simulink model "gate_V25_2016a"  (R2016a)
settings: Solver=FixedStepAuto  StartTime=0.0  StopTime=100  FixedStep=0.001  RelTol=1e-3
values from neighbouring files (symbols this model uses):
  CLOSE_CHAR = CHAR_STAR    (= 42)    [GateParameter.m]
  CLOSE_SIDE_VALUE = 2.95*oneSec    (= 2950)    [GateParameter.m]
  CLOSED = 12    [GateParameter.m]
  CLOSING = 13    [GateParameter.m]
  NO_PASS_ASSIG = 6    [GateParameter.m]
  OPEN = 14    [GateParameter.m]
  OPEN_CHAR = CHAR_HASH    (= 35)    [GateParameter.m]
  OPEN_SIDE_VALUE = 3*oneSec    (= 3000)    [GateParameter.m]
  OPEN_TIMEOUT = 60*oneSec    (= 60000)    [GateParameter.m]
  OPENING = 11    [GateParameter.m]
  OPENING_ACTIVE = 1    [GateParameter.m]
  PASS_ASSIGNED = 7    [GateParameter.m]
  PASS_INCOMPLETE = 8    [GateParameter.m]
  PASS_TIMEOUT = 10*oneSec    (= 10000)    [GateParameter.m]
  PASSWORD_VERIFIED = 5    [GateParameter.m]
  TIMEOUT = 9    [GateParameter.m]
  WRONG_PASSWORD = 2    [GateParameter.m]
undefined symbols (not defined in the file or in its folder): sigbuilder_block
libraries: simulink x9, arduinolib x4
(part 2 of 3)

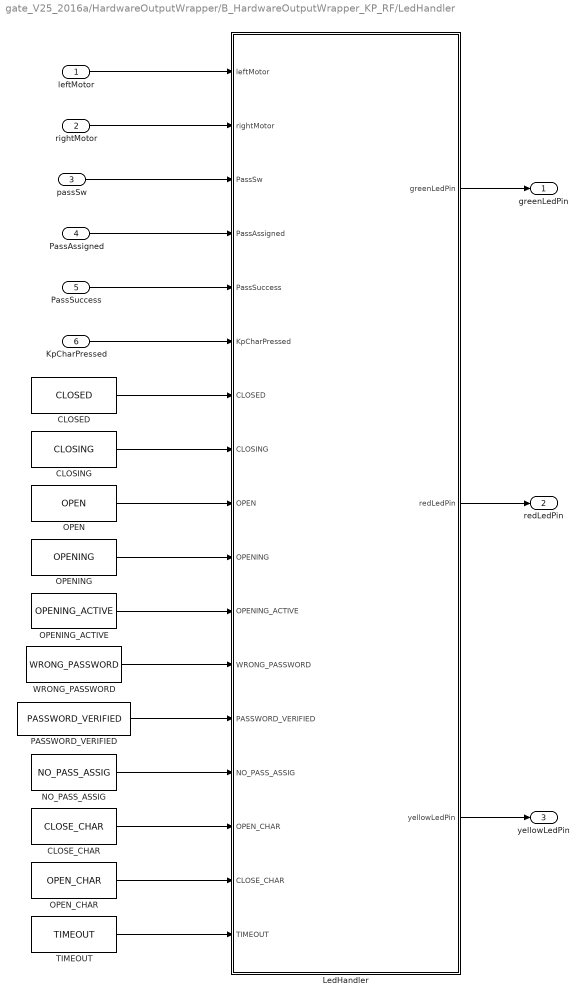
== system gate_V25_2016a/HardwareOutputWrapper/B_HardwareOutputWrapper_KP_RF/LedHandler ==
  leftMotor : Inport
  rightMotor : Inport  Port=2
  passSw : Inport  Port=3
  PassAssigned : Inport  Port=4
  PassSuccess : Inport  Port=5
  KpCharPressed : Inport  Port=6
  CLOSED : Constant  Value=CLOSED  SampleTime=-1
  CLOSE_CHAR : Constant  Value=CLOSE_CHAR  SampleTime=-1
  CLOSING : Constant  Value=CLOSING  SampleTime=-1
  LedHandler : Stateflow chart  TreatAsAtomicUnit=on
      settings: PermitHierarchicalResolution=ParametersOnly
  NO_PASS_ASSIG : Constant  Value=NO_PASS_ASSIG  SampleTime=-1
  OPEN : Constant  Value=OPEN  SampleTime=-1
  OPENING : Constant  Value=OPENING  SampleTime=-1
  OPENING_ACTIVE : Constant  Value=OPENING_ACTIVE  SampleTime=-1
  OPEN_CHAR : Constant  Value=OPEN_CHAR  SampleTime=-1
  PASSWORD_VERIFIED : Constant  Value=PASSWORD_VERIFIED  SampleTime=-1
  TIMEOUT : Constant  Value=TIMEOUT  SampleTime=-1
  WRONG_PASSWORD : Constant  Value=WRONG_PASSWORD  SampleTime=-1
  greenLedPin : Outport
  redLedPin : Outport  Port=2
  yellowLedPin : Outport  Port=3
  wires:
  TIMEOUT/1 -> LedHandler/17(TIMEOUT)
  OPEN_CHAR/1 -> LedHandler/16(CLOSE_CHAR)
  CLOSE_CHAR/1 -> LedHandler/15(OPEN_CHAR)
  KpCharPressed/1 -> LedHandler/6(KpCharPressed)
  NO_PASS_ASSIG/1 -> LedHandler/14(NO_PASS_ASSIG)
  PASSWORD_VERIFIED/1 -> LedHandler/13(PASSWORD_VERIFIED)
  WRONG_PASSWORD/1 -> LedHandler/12(WRONG_PASSWORD)
  OPENING_ACTIVE/1 -> LedHandler/11(OPENING_ACTIVE)
  CLOSED/1 -> LedHandler/7(CLOSED)
  CLOSING/1 -> LedHandler/8(CLOSING)
  OPEN/1 -> LedHandler/9(OPEN)
  OPENING/1 -> LedHandler/10(OPENING)
  PassSuccess/1 -> LedHandler/5(PassSuccess)
  PassAssigned/1 -> LedHandler/4(PassAssigned)
  passSw/1 -> LedHandler/3(PassSw)
  LedHandler/3(yellowLedPin) -> yellowLedPin/1
  LedHandler/2(redLedPin) -> redLedPin/1
  LedHandler/1(greenLedPin) -> greenLedPin/1
  rightMotor/1 -> LedHandler/2(rightMotor)
  leftMotor/1 -> LedHandler/1(leftMotor)

== system gate_V25_2016a/HardwareOutputWrapper/B_HardwareOutputWrapper_KP_RF/MotorHandler ==
  leftMotor : Inport
  rightMotor : Inport  Port=2
  CLOSED : Constant  Value=CLOSED  SampleTime=-1
  CLOSING : Constant  Value=CLOSING  SampleTime=-1
  MotorsHandler : Stateflow chart  TreatAsAtomicUnit=on
      settings: PermitHierarchicalResolution=ParametersOnly
  OPEN : Constant  Value=OPEN  SampleTime=-1
  OPENING : Constant  Value=OPENING  SampleTime=-1
  Unit Delay : UnitDelay  SampleTime=-1
  Unit Delay1 : UnitDelay  SampleTime=-1
  LeftPin : Outport
  ComPin : Outport  Port=2
  RightPin : Outport  Port=3
  wires:
  MotorsHandler/3(RightPin) -> RightPin/1
  MotorsHandler/2(ComPin) -> ComPin/1
  MotorsHandler/1(LeftPin) -> LeftPin/1
  OPENING/1 -> MotorsHandler/8(OPENING)
  OPEN/1 -> MotorsHandler/7(OPEN)
  CLOSING/1 -> MotorsHandler/6(CLOSING)
  CLOSED/1 -> MotorsHandler/5(CLOSED)
  Unit Delay1/1 -> MotorsHandler/4(oldRight)
  rightMotor/1 -> MotorsHandler/3(rightMotor), Unit Delay1/1
  Unit Delay/1 -> MotorsHandler/2(oldLeft)
  leftMotor/1 -> MotorsHandler/1(leftMotor), Unit Delay/1

== system gate_V25_2016a/HardwareOutputWrapper/C_HardwareOutputWrapper_RF/BulbHandler ==
  bulb : Inport
  bulbPin : Outport
  wires:
  bulb/1 -> bulbPin/1

== system gate_V25_2016a/HardwareOutputWrapper/C_HardwareOutputWrapper_RF/MotorHandler ==
  leftMotor : Inport
  rightMotor : Inport  Port=2
  CLOSED : Constant  Value=CLOSED  SampleTime=-1
  CLOSING : Constant  Value=CLOSING  SampleTime=-1
  MotorsHandler : Stateflow chart  TreatAsAtomicUnit=on
      settings: PermitHierarchicalResolution=ParametersOnly
  OPEN : Constant  Value=OPEN  SampleTime=-1
  OPENING : Constant  Value=OPENING  SampleTime=-1
  Unit Delay : UnitDelay  SampleTime=-1
  Unit Delay1 : UnitDelay  SampleTime=-1
  LeftPin : Outport
  ComPin : Outport  Port=2
  RightPin : Outport  Port=3
  wires:
  leftMotor/1 -> Unit Delay/1, MotorsHandler/1(leftMotor)
  Unit Delay/1 -> MotorsHandler/2(oldLeft)
  rightMotor/1 -> Unit Delay1/1, MotorsHandler/3(rightMotor)
  Unit Delay1/1 -> MotorsHandler/4(oldRight)
  CLOSED/1 -> MotorsHandler/5(CLOSED)
  CLOSING/1 -> MotorsHandler/6(CLOSING)
  OPEN/1 -> MotorsHandler/7(OPEN)
  OPENING/1 -> MotorsHandler/8(OPENING)
  MotorsHandler/1(LeftPin) -> LeftPin/1
  MotorsHandler/2(ComPin) -> ComPin/1
  MotorsHandler/3(RightPin) -> RightPin/1

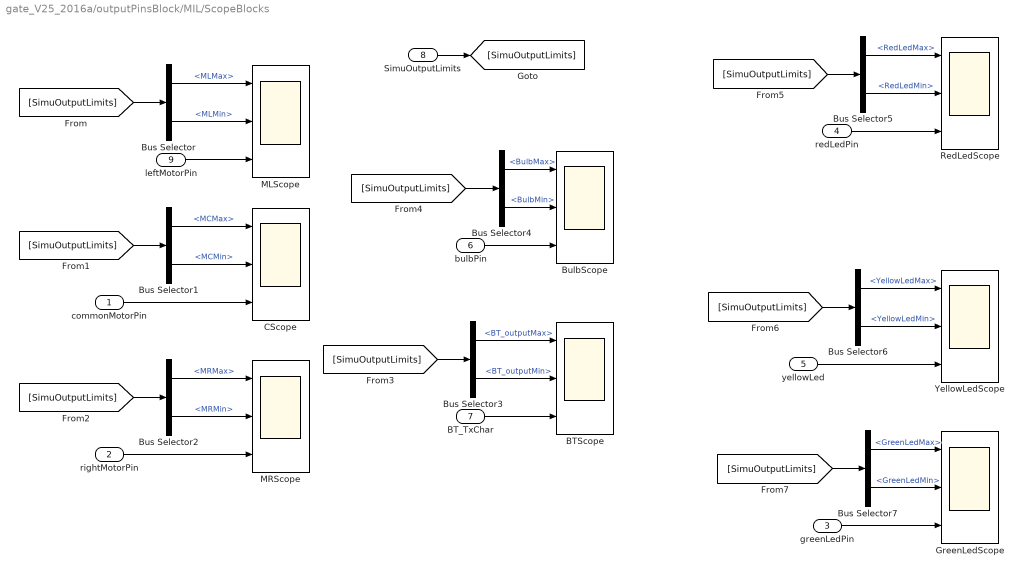
== system gate_V25_2016a/outputPinsBlock/MIL/ScopeBlocks ==
  commonMotorPin : Inport
  rightMotorPin : Inport  Port=2
  greenLedPin : Inport  Port=3
  redLedPin : Inport  Port=4
  yellowLed : Inport  Port=5
  bulbPin : Inport  Port=6
  BT_TxChar : Inport  Port=7
  SimuOutputLimits : Inport  Port=8
  leftMotorPin : Inport  Port=9
  BTScope : Scope  NumInputPorts=3
  BulbScope : Scope  NumInputPorts=3
  Bus Selector : BusSelector  OutputSignals=MLMax,MLMin
  Bus Selector1 : BusSelector  OutputSignals=MCMax,MCMin
  Bus Selector2 : BusSelector  OutputSignals=MRMax,MRMin
  Bus Selector3 : BusSelector  OutputSignals=BT_outputMax,BT_outputMin
  Bus Selector4 : BusSelector  OutputSignals=BulbMax,BulbMin
  Bus Selector5 : BusSelector  OutputSignals=RedLedMax,RedLedMin
  Bus Selector6 : BusSelector  OutputSignals=YellowLedMax,YellowLedMin
  Bus Selector7 : BusSelector  OutputSignals=GreenLedMax,GreenLedMin
  CScope : Scope  NumInputPorts=3
  GreenLedScope : Scope  NumInputPorts=3
  MLScope : Scope  NumInputPorts=3
  MRScope : Scope  NumInputPorts=3
  RedLedScope : Scope  NumInputPorts=3
  YellowLedScope : Scope  NumInputPorts=3
  wires:
  rightMotorPin/1 -> MRScope/3
  commonMotorPin/1 -> CScope/3
  bulbPin/1 -> BulbScope/3
  greenLedPin/1 -> GreenLedScope/3
  yellowLed/1 -> YellowLedScope/3
  redLedPin/1 -> RedLedScope/3
  BT_TxChar/1 -> BTScope/3
  SimuOutputLimits/1 -> [SimuOutputLimits]
  [SimuOutputLimits] -> Bus Selector/1
  leftMotorPin/1 -> MLScope/3
  Bus Selector/1 -> MLScope/1  "<MLMax>"
  Bus Selector/2 -> MLScope/2  "<MLMin>"
  [SimuOutputLimits] -> Bus Selector1/1
  Bus Selector1/1 -> CScope/1  "<MCMax>"
  Bus Selector1/2 -> CScope/2  "<MCMin>"
  [SimuOutputLimits] -> Bus Selector2/1
  Bus Selector2/1 -> MRScope/1  "<MRMax>"
  Bus Selector2/2 -> MRScope/2  "<MRMin>"
  [SimuOutputLimits] -> Bus Selector3/1
  Bus Selector3/1 -> BTScope/1  "<BT_outputMax>"
  Bus Selector3/2 -> BTScope/2  "<BT_outputMin>"
  [SimuOutputLimits] -> Bus Selector4/1
  Bus Selector4/1 -> BulbScope/1  "<BulbMax>"
  Bus Selector4/2 -> BulbScope/2  "<BulbMin>"
  [SimuOutputLimits] -> Bus Selector5/1
  Bus Selector5/1 -> RedLedScope/1  "<RedLedMax>"
  Bus Selector5/2 -> RedLedScope/2  "<RedLedMin>"
  [SimuOutputLimits] -> Bus Selector6/1
  Bus Selector6/1 -> YellowLedScope/1  "<YellowLedMax>"
  Bus Selector6/2 -> YellowLedScope/2  "<YellowLedMin>"
  [SimuOutputLimits] -> Bus Selector7/1
  Bus Selector7/1 -> GreenLedScope/1  "<GreenLedMax>"
  Bus Selector7/2 -> GreenLedScope/2  "<GreenLedMin>"

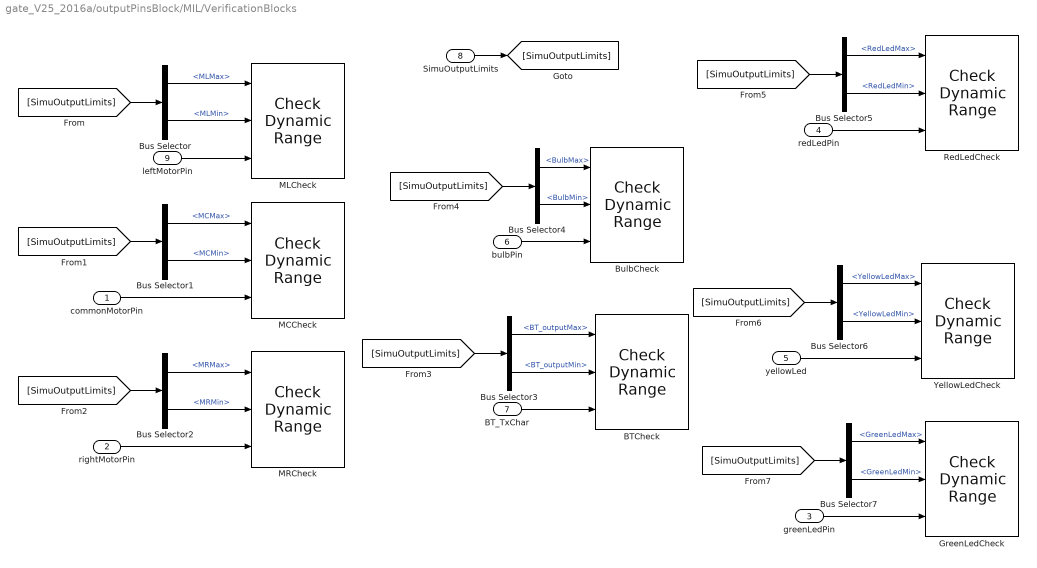
== system gate_V25_2016a/outputPinsBlock/MIL/VerificationBlocks  ==
  commonMotorPin : Inport
  rightMotorPin : Inport  Port=2
  greenLedPin : Inport  Port=3
  redLedPin : Inport  Port=4
  yellowLed : Inport  Port=5
  bulbPin : Inport  Port=6
  BT_TxChar : Inport  Port=7
  SimuOutputLimits : Inport  Port=8
  leftMotorPin : Inport  Port=9
  BTCheck : simulink/Model Verification/Check  Dynamic Range  Description=min < sig < max  enabled=on  stopWhenAssertionFail=on  export=off  icon=graphic
  BulbCheck : simulink/Model Verification/Check  Dynamic Range  Description=min < sig < max  enabled=on  stopWhenAssertionFail=on  export=off  icon=graphic
  Bus Selector : BusSelector  OutputSignals=MLMax,MLMin
  Bus Selector1 : BusSelector  OutputSignals=MCMax,MCMin
  Bus Selector2 : BusSelector  OutputSignals=MRMax,MRMin
  Bus Selector3 : BusSelector  OutputSignals=BT_outputMax,BT_outputMin
  Bus Selector4 : BusSelector  OutputSignals=BulbMax,BulbMin
  Bus Selector5 : BusSelector  OutputSignals=RedLedMax,RedLedMin
  Bus Selector6 : BusSelector  OutputSignals=YellowLedMax,YellowLedMin
  Bus Selector7 : BusSelector  OutputSignals=GreenLedMax,GreenLedMin
  GreenLedCheck : simulink/Model Verification/Check  Dynamic Range  Description=min < sig < max  enabled=on  stopWhenAssertionFail=on  export=off  icon=graphic
  MCCheck : simulink/Model Verification/Check  Dynamic Range  Description=min < sig < max  enabled=on  stopWhenAssertionFail=on  export=off  icon=graphic
  MLCheck : simulink/Model Verification/Check  Dynamic Range  Description=min < sig < max  enabled=on  stopWhenAssertionFail=on  export=off  icon=graphic
  MRCheck : simulink/Model Verification/Check  Dynamic Range  Description=min < sig < max  enabled=on  stopWhenAssertionFail=on  export=off  icon=graphic
  RedLedCheck : simulink/Model Verification/Check  Dynamic Range  Description=min < sig < max  enabled=on  stopWhenAssertionFail=on  export=off  icon=graphic
  YellowLedCheck : simulink/Model Verification/Check  Dynamic Range  Description=min < sig < max  enabled=on  stopWhenAssertionFail=on  export=off  icon=graphic
  wires:
  rightMotorPin/1 -> MRCheck/3
  commonMotorPin/1 -> MCCheck/3
  bulbPin/1 -> BulbCheck/3
  greenLedPin/1 -> GreenLedCheck/3
  yellowLed/1 -> YellowLedCheck/3
  redLedPin/1 -> RedLedCheck/3
  BT_TxChar/1 -> BTCheck/3
  SimuOutputLimits/1 -> [SimuOutputLimits]
  [SimuOutputLimits] -> Bus Selector/1
  leftMotorPin/1 -> MLCheck/3
  Bus Selector/1 -> MLCheck/1  "<MLMax>"
  Bus Selector/2 -> MLCheck/2  "<MLMin>"
  [SimuOutputLimits] -> Bus Selector1/1
  Bus Selector1/1 -> MCCheck/1  "<MCMax>"
  Bus Selector1/2 -> MCCheck/2  "<MCMin>"
  [SimuOutputLimits] -> Bus Selector2/1
  Bus Selector2/1 -> MRCheck/1  "<MRMax>"
  Bus Selector2/2 -> MRCheck/2  "<MRMin>"
  [SimuOutputLimits] -> Bus Selector3/1
  Bus Selector3/1 -> BTCheck/1  "<BT_outputMax>"
  Bus Selector3/2 -> BTCheck/2  "<BT_outputMin>"
  [SimuOutputLimits] -> Bus Selector4/1
  Bus Selector4/1 -> BulbCheck/1  "<BulbMax>"
  Bus Selector4/2 -> BulbCheck/2  "<BulbMin>"
  [SimuOutputLimits] -> Bus Selector5/1
  Bus Selector5/1 -> RedLedCheck/1  "<RedLedMax>"
  Bus Selector5/2 -> RedLedCheck/2  "<RedLedMin>"
  [SimuOutputLimits] -> Bus Selector6/1
  Bus Selector6/1 -> YellowLedCheck/1  "<YellowLedMax>"
  Bus Selector6/2 -> YellowLedCheck/2  "<YellowLedMin>"
  [SimuOutputLimits] -> Bus Selector7/1
  Bus Selector7/1 -> GreenLedCheck/1  "<GreenLedMax>"
  Bus Selector7/2 -> GreenLedCheck/2  "<GreenLedMin>"

== stateflow chart gate_V25_2016a/GateLogic/A_Variant_BT_KP_RF/GateLogicStatemachine ==
  state opening
    entry:
    bulb = true;
    state openLeftSide
      entry:
      leftMotor = OPENING;
      openSideDelay = 0;
      during:
      openSideDelay++;
    state openRightSide
      entry:
      rightMotor = OPENING;
    (default) -> openLeftSide
    openLeftSide -> openRightSide : [openSideDelay == OPEN_SIDE_VALUE]
  state init
    entry:
    passSuccess = NO_PASS_ASSIG;
    gotoReady = false;
    bulb = 0;
    leftMotor = CLOSED;
    rightMotor = CLOSED;
    state AssignPass
      entry:
      counter = 0;
      state addToPass
        entry:
        password[counter] = KpCharPressed;
      state MonitoringNumber
      state PassAssigned
        entry:
        gotoReady = true;
      (junction 259) -> addToPass : [KpCharPressed != 0]
      MonitoringNumber -> (junction 259) [order 1] : [hasChanged(KpCharPressed)]
      (default) -> MonitoringNumber
      addToPass -> MonitoringNumber [order 1] : [counter < 5]/counter++;
      MonitoringNumber -> PassAssigned [order 2] : [RfOpen == true]
      addToPass -> PassAssigned [order 2] : [counter == 5]
          | / passAssigned = true;...
          | passSuccess = PASS_ASSIGNED;
    state idle
      entry:
      passAssigned = false;
    state PassAssignedPreviously
      entry:
      password[0] = passwordIn[0];
      password[1] = passwordIn[1];
      password[2] = passwordIn[2];
      password[3] = passwordIn[3];
      password[4] = passwordIn[4];
      password[5] = passwordIn[5];
      passAssigned = passAssignedIn;
      gotoReady = true;
    (default) -> idle
    idle -> AssignPass [order 1] : [passSwitch==true]
    idle -> PassAssignedPreviously [order 2] : [passAssignedIn]
    AssignPass -> idle : [passSwitch==false]
  state ready
    entry:
    bulb = false;
    leftMotor = CLOSED;
    rightMotor = CLOSED;
    openingActive = 0;
    state BTPassHandler
      state monitorBtnPressed
      state btnPressed
        entry:
        trialPass[counter] = BtCharReceived;
      state initTrailPass
        entry:
        initCounter = 1;
        state initiatePass
          entry:
          trialPass[initCounter] = 0;
        (junction 295) -> ready.BTPassHandler.initTrailPass.initiatePass
        (default) -> (junction 295)
        ready.BTPassHandler.initTrailPass.initiatePass -> (junction 295) : [initCounter < 5]...
            | /initCounter++;
      state verifyPass
        (default) -> (junction 301)
        (junction 301) -> (junction 302) [order 1] : [trialPass[0] != password[0]]
        (junction 301) -> (junction 303) [order 2]
        (junction 302) -> (junction 319) : {passSuccess = WRONG_PASSWORD;}
        (junction 303) -> (junction 304) [order 1] : [trialPass[1] != password[1]]
        (junction 303) -> (junction 305) [order 2]
        (junction 304) -> (junction 318) : {passSuccess = WRONG_PASSWORD;}
        (junction 305) -> (junction 306) [order 1] : [trialPass[2] != password[2]]
        (junction 305) -> (junction 307) [order 2]
        (junction 306) -> (junction 317) : {passSuccess = WRONG_PASSWORD;}
        (junction 307) -> (junction 308) [order 1] : [trialPass[3] != password[3]]
        (junction 307) -> (junction 309) [order 2]
        (junction 308) -> (junction 316) : {passSuccess = WRONG_PASSWORD;}
        (junction 309) -> (junction 310) [order 1] : [trialPass[4] != password[4]]
        (junction 309) -> (junction 311) [order 2]
        (junction 310) -> (junction 315) : {passSuccess = WRONG_PASSWORD;}
        (junction 311) -> (junction 312) [order 1] : [trialPass[5] != password[5]]
        (junction 311) -> (junction 313) [order 2] : {passSuccess = PASSWORD_VERIFIED;}
        (junction 312) -> (junction 314) : {passSuccess = WRONG_PASSWORD;}
        (junction 314) -> (junction 313)
        (junction 315) -> (junction 314)
        (junction 316) -> (junction 315)
        (junction 317) -> (junction 316)
        (junction 318) -> (junction 317)
        (junction 319) -> (junction 318)
        (junction 313) -> (junction 320)
      (default) -> ready.BTPassHandler.initTrailPass
      ready.BTPassHandler.monitorBtnPressed -> (junction 277) : [hasChanged...
          | (BtCharReceived)]
      (junction 277) -> ready.BTPassHandler.btnPressed : [BtCharReceived != 0]/{counter++;}
      ready.BTPassHandler.initTrailPass -> ready.BTPassHandler.monitorBtnPressed : [initCounter == 5]...
          | /{counter = 0;}
      ready.BTPassHandler.btnPressed -> ready.BTPassHandler.monitorBtnPressed [order 1] : [counter < 5]
      (junction 279) -> ready.BTPassHandler.initTrailPass
      ready.BTPassHandler.btnPressed -> ready.BTPassHandler.verifyPass [order 2] : [counter >= 5]
      ready.BTPassHandler.verifyPass -> (junction 279) : [(passSuccess == PASSWORD_VERIFIED)]
          | / {openingActive = OPENING_ACTIVE;}
    state openingGate
    state MonitorInput
      entry:
      passTimer = 0;
    state KpPassHandler
      du:
      passTimer++;
      state monitorBtnPressed
      state btnPressed
        entry:
        trialPass[counter] = KpCharPressed;
      state initTrailPass
        entry:
        initCounter = 1;
        state initiatePass
          entry:
          trialPass[initCounter] = 0;
        (junction 269) -> ready.KpPassHandler.initTrailPass.initiatePass
        (default) -> (junction 269)
        ready.KpPassHandler.initTrailPass.initiatePass -> (junction 269) : [initCounter < 5]...
            | /initCounter++;
      state verifyPass
        (default) -> (junction 115)
        (junction 115) -> (junction 116) [order 1] : [trialPass[0] != password[0]]
        (junction 115) -> (junction 119) [order 2]
        (junction 116) -> (junction 118) : {passSuccess = WRONG_PASSWORD;}
        (junction 119) -> (junction 122) [order 1] : [trialPass[1] != password[1]]
        (junction 119) -> (junction 120) [order 2]
        (junction 122) -> (junction 121) : {passSuccess = WRONG_PASSWORD;}
        (junction 120) -> (junction 144) [order 1] : [trialPass[2] != password[2]]
        (junction 120) -> (junction 143) [order 2]
        (junction 144) -> (junction 168) : {passSuccess = WRONG_PASSWORD;}
        (junction 143) -> (junction 149) [order 1] : [trialPass[3] != password[3]]
        (junction 143) -> (junction 153) [order 2]
        (junction 149) -> (junction 169) : {passSuccess = WRONG_PASSWORD;}
        (junction 153) -> (junction 156) [order 1] : [trialPass[4] != password[4]]
        (junction 153) -> (junction 157) [order 2]
        (junction 156) -> (junction 170) : {passSuccess = WRONG_PASSWORD;}
        (junction 157) -> (junction 158) [order 1] : [trialPass[5] != password[5]]
        (junction 157) -> (junction 164) [order 2] : {passSuccess = PASSWORD_VERIFIED;}
        (junction 158) -> (junction 171) : {passSuccess = WRONG_PASSWORD;}
        (junction 171) -> (junction 164)
        (junction 170) -> (junction 171)
        (junction 169) -> (junction 170)
        (junction 168) -> (junction 169)
        (junction 121) -> (junction 168)
        (junction 118) -> (junction 121)
        (junction 164) -> (junction 165)
      (default) -> ready.KpPassHandler.initTrailPass
      ready.KpPassHandler.monitorBtnPressed -> (junction 263) : [hasChanged...
          | (KpCharPressed)]
      (junction 263) -> ready.KpPassHandler.btnPressed : [KpCharPressed != 0]/{counter++;}
      ready.KpPassHandler.initTrailPass -> ready.KpPassHandler.monitorBtnPressed : [initCounter == 5]...
          | /{counter = 0;}
      ready.KpPassHandler.btnPressed -> ready.KpPassHandler.monitorBtnPressed [order 1] : [counter < 5]
      (junction 262) -> ready.KpPassHandler.initTrailPass : [(KpCharPressed == OPEN_CHAR)...
          |  && (KpCharPressed != 0)]...
          |  / {openingActive = OPENING_ACTIVE;}
      ready.KpPassHandler.btnPressed -> ready.KpPassHandler.verifyPass [order 2] : [counter >= 5]
      ready.KpPassHandler.verifyPass -> (junction 262) : [hasChanged(KpCharPressed) && (passSuccess == PASSWORD_VERIFIED)]
    (junction 350) -> BTPassHandler : [(BtCharReceived != 0) ...
        | && passAssigned]
        | /passSuccess = PASS_INCOMPLETE;...
        | trialPass[0] = BtCharReceived;
    MonitorInput -> (junction 350) [order 3] : [hasChanged...
        | (BtCharReceived)]
    BTPassHandler -> openingGate [order 2] : [openingActive == OPENING_ACTIVE]
    BTPassHandler -> MonitorInput [order 1] : [passSuccess == WRONG_PASSWORD]
    MonitorInput -> openingGate [order 1] : [RfOpen]/{openingActive = OPENING_ACTIVE;}
    (default) -> MonitorInput
    KpPassHandler -> MonitorInput [order 3] : [(passTimer == PASS_TIMEOUT)]
        | /passSuccess = TIMEOUT;
    KpPassHandler -> openingGate [order 1] : [openingActive == OPENING_ACTIVE]
    MonitorInput -> (junction 260) [order 2] : [hasChanged...
        | (KpCharPressed)]
    KpPassHandler -> MonitorInput [order 2] : [(passSuccess == WRONG_PASSWORD)]
    (junction 260) -> KpPassHandler : [(KpCharPressed != 0) ...
        | &&(KpCharPressed != OPEN_CHAR)...
        | &&(KpCharPressed != CLOSE_CHAR)...
        | && passAssigned]
        | /passSuccess = PASS_INCOMPLETE;...
        | trialPass[0] = KpCharPressed;
  state closing
    state closingRightSide
      entry:
      rightMotor = CLOSING;
      closeSideDelay = 0;
      during:
      closeSideDelay++;
    state closingLeftSide
      entry:
      leftMotor = CLOSING;
    (default) -> closingRightSide
    closingRightSide -> closingLeftSide : [closeSideDelay == CLOSE_SIDE_VALUE]
  state open
    state gateOpen
      entry:
      closing_active = false;
      leftMotor = OPEN;
      rightMotor = OPEN;
      openTimer = 0;
      du:
      openTimer++;
    state closing
      entry:
      closing_active = true;
    (default) -> gateOpen
    gateOpen -> (junction 264) [order 1] : [hasChanged(KpCharPressed)]
    (junction 264) -> open.closing : [(KpCharPressed == CLOSE_CHAR)]
    gateOpen -> (junction 355) [order 3] : [hasChanged(BtCharReceived)]
    (junction 355) -> open.closing : [BtCharReceived == CLOSE_CHAR]
    gateOpen -> open.closing [order 2] : [RfClose]
    gateOpen -> open.closing [order 4] : [openTimer == OPEN_TIMEOUT]
  ready -> (junction 258) [order 1] : [hasChanged(passSwitch)]
  (junction 258) -> init : [passSwitch]
  (default) -> init
  init -> ready [order 1] : [gotoReady == true]
  ready -> opening [order 2] : [openingActive == OPENING_ACTIVE]
  init -> ready [order 2] : [RfOpen == true]
  closing -> ready : [(current_sensor == 0)...
      | &&(leftMotor == CLOSING)...
      | &&(rightMotor == CLOSING)]
  opening -> open : [(current_sensor == 0)...
      | && (leftMotor == OPENING)...
      | && (rightMotor == OPENING)]
  open -> closing : [closing_active == true]
  data: KpCharPressed input; RfOpen input; openingActive local uint8; passSwitch input; counter local uint8; closing_active local uint8; current_sensor input; initCounter local uint8; openSideDelay local uint16; leftMotor output uint8 =0; rightMotor output uint8 =0; bulb output boolean; RfClose input; closeSideDelay local uint16; BtCharReceived input; OPENING_ACTIVE input =2; WRONG_PASSWORD input =1; OPEN_SIDE_VALUE input =20; CLOSE_SIDE_VALUE input =20; OPEN_TIMEOUT input =999999; PASSWORD_VERIFIED input =3; CLOSE_CHAR input =12; OPEN_CHAR input; OPENING input =2; CLOSED input =1; CLOSING input =4; OPEN input =3; passAssigned output boolean; gotoReady local boolean; passSuccess output uint8 =0; NO_PASS_ASSIG input; PASS_ASSIGNED input; PASS_INCOMPLETE input; PASS_TIMEOUT input; passTimer local uint16; TIMEOUT input; openTimer local uint16; password output uint8 size=6; passwordIn input size=6; passAssignedIn input; trialPass output uint8 size=6

== stateflow chart gate_V25_2016a/HardwareOutputWrapper/A_HardwareOutputWrapper_BT_KP_RF/BT_TxHandler/BT_TxHandler ==
  state Idle
    entry:
    BT_TxChar = 0;
  state WrongPass
    entry:
    BT_TxChar = 119;
    counter = 0;
    du:
    counter++;
  state BtInput
  state sendClose
    entry:
    BT_TxChar = 99;
  state sendOpen
    entry:
    BT_TxChar = 98;
  state sendOpening
    entry:
    BT_TxChar = 97;
  (default) -> Idle
  Idle -> (junction 8) : [hasChanged(BTCharReceived)]
  (junction 8) -> BtInput : [BTCharReceived != 0]
  sendClose -> Idle : [leftMotor == CLOSED]
  WrongPass -> Idle : [counter >= 10]
  BtInput -> WrongPass [order 2] : [PassSuccess == WRONG_PASSWORD]
  BtInput -> sendOpening [order 1] : [leftMotor == OPENING]
  sendOpen -> sendClose : [rightMotor == CLOSING]
  sendOpening -> sendOpen : [rightMotor == OPEN]
  data: BTCharReceived input; leftMotor input; rightMotor input; BT_TxChar output uint8; PassSuccess input; CLOSED input; CLOSING input; OPEN input; OPENING input; WRONG_PASSWORD input; counter local uint8

== stateflow chart gate_V25_2016a/HardwareOutputWrapper/A_HardwareOutputWrapper_BT_KP_RF/LedHandler/LedHandler ==
  state AssigningPass
    en:
    counter = 0;
    state Start
      en:
      yellowLedPin = true;
      greenLedPin = false;
      redLedPin = false;
    state correctPassAssigned
      du:
      counter++;
    state incorrectPassAssigned
      du:
      counter++;
    (default) -> AssigningPass.Start
    AssigningPass.Start -> correctPassAssigned [order 1] : [PassAssigned == true]/greenLedPin = true;
    AssigningPass.Start -> incorrectPassAssigned [order 2] : [(PassSw == false) && (PassAssigned == false)]
        | /redLedPin = true;...
        | yellowLedPin = false;
    correctPassAssigned -> correctPassAssigned : [(hasChanged(PassSw)) ...
        | && (PassSw == false)]
        | /yellowLedPin = false;
  state EnteringPass
    en:
    counter = 0;
    state correctPass
      en:
      yellowLedPin = false;
      greenLedPin = true;
      redLedPin = false;
      du:
      counter++;
    state Start
    state IncorrectPass
      en:
      yellowLedPin = false;
      greenLedPin = false;
      redLedPin = true;
      du:
      counter++;
    EnteringPass.Start -> correctPass [order 1] : [PassSuccess == PASSWORD_VERIFIED]
    (default) -> EnteringPass.Start
    EnteringPass.Start -> IncorrectPass [order 2] : [(PassSuccess == TIMEOUT)...
        |  || (PassSuccess == WRONG_PASSWORD)]
  state Idle
    en:
    yellowLedPin = false;
    greenLedPin = false;
    redLedPin = false;
  state GateOn
    en:
    yellowLedPin = false;
    greenLedPin = true;
    redLedPin = false;
  (default) -> Idle
  EnteringPass -> Idle [order 2] : [PassSuccess == NO_PASS_ASSIG]
  Idle -> AssigningPass [order 1] : [PassSw == true]
  correctPass -> Idle : [counter >= 4800]
  AssigningPass -> Idle [order 1] : [(counter >= 4900)]
  Idle -> EnteringPass [order 2] : [(hasChanged(KpCharPressed)) ...
      | && (KpCharPressed != 0)...
      | && (KpCharPressed != OPEN_CHAR)...
      | && (KpCharPressed != CLOSE_CHAR)...
      | && (PassAssigned == true)]
      | /yellowLedPin = true;
  IncorrectPass -> Idle : [counter >= 4800]
  Idle -> GateOn [order 3] : [(leftMotor == OPENING)...
      |  || (leftMotor == OPEN)...
      |  || (leftMotor == CLOSING)]
  GateOn -> Idle : [leftMotor == CLOSED]
  EnteringPass -> GateOn [order 1] : [(leftMotor == OPENING)...
      | || (leftMotor == OPEN)...
      | || (leftMotor == CLOSING)]
  AssigningPass -> GateOn [order 2] : [(leftMotor == OPENING)...
      |  || (leftMotor == OPEN)...
      |  || (leftMotor == CLOSING)]
  data: leftMotor input; rightMotor input; greenLedPin output boolean =false; redLedPin output boolean =false; yellowLedPin output boolean =false; PassSw input; counter local uint16; PassAssigned input; PassSuccess input; KpCharPressed input; CLOSED input; CLOSING input; OPEN input; OPENING input; OPENING_ACTIVE input; WRONG_PASSWORD input; PASSWORD_VERIFIED input; NO_PASS_ASSIG input; OPEN_CHAR input; CLOSE_CHAR input; TIMEOUT input

== stateflow chart gate_V25_2016a/GateLogic/B_Variant_KP_RF/GateLogicStatemachine ==
  state opening
    entry:
    bulb = true;
    state openLeftSide
      entry:
      leftMotor = OPENING;
      openSideDelay = 0;
      during:
      openSideDelay++;
    state openRightSide
      entry:
      rightMotor = OPENING;
    (default) -> openLeftSide
    openLeftSide -> openRightSide : [openSideDelay == OPEN_SIDE_VALUE]
  state init
    entry:
    passSuccess = NO_PASS_ASSIG;
    gotoReady = false;
    bulb = 0;
    leftMotor = CLOSED;
    rightMotor = CLOSED;
    state AssignPass
      entry:
      counter = 0;
      password[0] = 0;
      password[1] = 0;
      password[2] = 0;
      password[3] = 0;
      password[4] = 0;
      password[5] = 0;
      state addToPass
        entry:
        password[counter] = KpCharPressed;
      state MonitoringNumber
      state PassAssigned
        entry:
        gotoReady = true;
      MonitoringNumber -> (junction 259) [order 1] : [hasChanged(KpCharPressed)]
      (junction 259) -> addToPass : [KpCharPressed != 0]
      (default) -> MonitoringNumber
      addToPass -> MonitoringNumber [order 1] : [counter < 5]/counter++;
      addToPass -> PassAssigned [order 2] : [counter == 5]
          | / passAssigned = true;...
          | passSuccess = PASS_ASSIGNED;
      MonitoringNumber -> PassAssigned [order 2] : [RfOpen == true]
    state idle
      entry:
      passAssigned = false;
    state PassAssignedPreviously
      entry:
      password[0] = passwordIn[0];
      password[1] = passwordIn[1];
      password[2] = passwordIn[2];
      password[3] = passwordIn[3];
      password[4] = passwordIn[4];
      password[5] = passwordIn[5];
      passAssigned = passAssignedIn;
      gotoReady = true;
    (default) -> idle
    idle -> AssignPass [order 1] : [passSwitch==true]
    idle -> PassAssignedPreviously [order 2] : [passAssignedIn]
    AssignPass -> idle : [passSwitch==false]
  state ready
    entry:
    bulb = false;
    leftMotor = CLOSED;
    rightMotor = CLOSED;
    openingActive = 0;
    state openingGate
    state MonitorInput
      entry:
      passTimer = 0;
    state KpPassHandler
      du:
      passTimer++;
      state monitorBtnPressed
      state btnPressed
        entry:
        trialPass[counter] = KpCharPressed;
      state initTrailPass
        entry:
        initCounter = 1;
        state initiatePass
          entry:
          trialPass[initCounter] = 0;
        (junction 269) -> initiatePass
        (default) -> (junction 269)
        initiatePass -> (junction 269) : [initCounter < 5]...
            | /initCounter++;
      state verifyPass
        (default) -> (junction 115)
        (junction 115) -> (junction 116) [order 1] : [trialPass[0] != password[0]]
        (junction 115) -> (junction 119) [order 2]
        (junction 116) -> (junction 118) : {passSuccess = WRONG_PASSWORD;}
        (junction 119) -> (junction 122) [order 1] : [trialPass[1] != password[1]]
        (junction 119) -> (junction 120) [order 2]
        (junction 122) -> (junction 121) : {passSuccess = WRONG_PASSWORD;}
        (junction 120) -> (junction 144) [order 1] : [trialPass[2] != password[2]]
        (junction 120) -> (junction 143) [order 2]
        (junction 144) -> (junction 168) : {passSuccess = WRONG_PASSWORD;}
        (junction 143) -> (junction 149) [order 1] : [trialPass[3] != password[3]]
        (junction 143) -> (junction 153) [order 2]
        (junction 149) -> (junction 169) : {passSuccess = WRONG_PASSWORD;}
        (junction 153) -> (junction 156) [order 1] : [trialPass[4] != password[4]]
        (junction 153) -> (junction 157) [order 2]
        (junction 156) -> (junction 170) : {passSuccess = WRONG_PASSWORD;}
        (junction 157) -> (junction 158) [order 1] : [trialPass[5] != password[5]]
        (junction 157) -> (junction 164) [order 2] : {passSuccess = PASSWORD_VERIFIED;}
        (junction 158) -> (junction 171) : {passSuccess = WRONG_PASSWORD;}
        (junction 171) -> (junction 164)
        (junction 170) -> (junction 171)
        (junction 169) -> (junction 170)
        (junction 168) -> (junction 169)
        (junction 121) -> (junction 168)
        (junction 118) -> (junction 121)
        (junction 164) -> (junction 165)
      (default) -> initTrailPass
      monitorBtnPressed -> (junction 263) : [hasChanged...
          | (KpCharPressed)]
      (junction 263) -> btnPressed : [KpCharPressed != 0]/{counter++;}
      initTrailPass -> monitorBtnPressed : [initCounter == 5]...
          | /{counter = 0;}
      btnPressed -> monitorBtnPressed [order 1] : [counter < 5]
      (junction 262) -> initTrailPass : [(KpCharPressed == OPEN_CHAR)...
          |  && (KpCharPressed != 0)]...
          |  / {openingActive = OPENING_ACTIVE;}
      btnPressed -> verifyPass [order 2] : [counter >= 5]
      verifyPass -> (junction 262) : [hasChanged(KpCharPressed) && (passSuccess == PASSWORD_VERIFIED)]
    (default) -> MonitorInput
    MonitorInput -> openingGate [order 1] : [RfOpen]/{openingActive = OPENING_ACTIVE;}
    KpPassHandler -> MonitorInput [order 3] : [(passTimer == PASS_TIMEOUT)]
        | /passSuccess = TIMEOUT;
    KpPassHandler -> openingGate [order 1] : [openingActive == OPENING_ACTIVE]
    MonitorInput -> (junction 260) [order 2] : [hasChanged...
        | (KpCharPressed)]
    KpPassHandler -> MonitorInput [order 2] : [(passSuccess == WRONG_PASSWORD)]
    (junction 260) -> KpPassHandler : [(KpCharPressed != 0) ...
        | &&(KpCharPressed != OPEN_CHAR)...
        | &&(KpCharPressed != CLOSE_CHAR)...
        | && passAssigned]
        | /passSuccess = PASS_INCOMPLETE;...
        | trialPass[0] = KpCharPressed;
  state closing
    state closingRightSide
      entry:
      rightMotor = CLOSING;
      closeSideDelay = 0;
      during:
      closeSideDelay++;
    state closingLeftSide
      entry:
      leftMotor = CLOSING;
    (default) -> closingRightSide
    closingRightSide -> closingLeftSide : [closeSideDelay == CLOSE_SIDE_VALUE]
  state open
    state gateOpen
      entry:
      closing_active = false;
      leftMotor = OPEN;
      rightMotor = OPEN;
      openTimer = 0;
      du:
      openTimer++;
    state closing
      entry:
      closing_active = true;
    (default) -> gateOpen
    gateOpen -> (junction 264) [order 1] : [hasChanged(KpCharPressed)]
    (junction 264) -> open.closing : [(KpCharPressed == CLOSE_CHAR)]
    gateOpen -> open.closing [order 2] : [RfClose]
    gateOpen -> open.closing [order 3] : [openTimer == OPEN_TIMEOUT]
  ready -> (junction 258) [order 1] : [hasChanged(passSwitch)]
  (junction 258) -> init : [passSwitch]
  (default) -> init
  init -> ready [order 1] : [gotoReady == true]
  ready -> opening [order 2] : [openingActive == OPENING_ACTIVE]
  init -> ready [order 2] : [RfOpen == true]
  closing -> ready : [(current_sensor == 0)...
      | &&(leftMotor == CLOSING)...
      | &&(rightMotor == CLOSING)]
  opening -> open : [(current_sensor == 0)...
      | && (leftMotor == OPENING)...
      | && (rightMotor == OPENING)]
  open -> closing : [closing_active == true]
  data: KpCharPressed input; RfOpen input; openingActive local uint8; passSwitch input; trialPass local uint8 size=6; counter local uint8; closing_active local uint8; current_sensor input; initCounter local uint8; openSideDelay local uint16; leftMotor output uint8 =0; rightMotor output uint8 =0; bulb output boolean; RfClose input; closeSideDelay local uint16; OPENING_ACTIVE input =2; WRONG_PASSWORD input =1; OPEN_SIDE_VALUE input =20; CLOSE_SIDE_VALUE input =20; OPEN_TIMEOUT input =999999; PASSWORD_VERIFIED input =3; CLOSE_CHAR input =12; OPEN_CHAR input; OPENING input =2; CLOSED input =1; CLOSING input =4; OPEN input =3; passAssigned output boolean; gotoReady local boolean; passSuccess output uint8 =0; NO_PASS_ASSIG input; PASS_ASSIGNED input; PASS_INCOMPLETE input; PASS_TIMEOUT input; passTimer local uint16; TIMEOUT input; openTimer local uint16; password output uint8 size=6; passwordIn input size=6; passAssignedIn input

== stateflow chart gate_V25_2016a/RFHandler/RFHandlerL ==
  state Close
    entry:
    RFOpen = false;
    RFClose = true;
  state RFOff
    entry:
    RFOpen = false;
    RFClose = false;
  state Open
    entry:
    RFOpen = true;
    RFClose = false;
    counter = 0;
    du:
    counter++;
  Close -> RFOff [order 1] : [rightMotor == CLOSED]
  Close -> (junction 11) [order 2] : [hasChanged(btn)]
  (junction 11) -> Close [order 2] : [(btn == 1) ...
      | && ((leftMotor == OPENING)...
      | || (leftMotor == OPEN))]
  (default) -> RFOff
  RFOff -> (junction 11) : [hasChanged(btn)]
  Open -> (junction 11) [order 2] : [hasChanged(btn)]
  (junction 11) -> Open [order 1] : [(btn == 1) ...
      | && ((leftMotor == CLOSING)...
      | || (leftMotor == CLOSED))]
  Open -> RFOff [order 1] : [(counter == 5) ...
      | && ((leftMotor == CLOSING)...
      | || (leftMotor == CLOSED))]
  data: btn input; RFClose output boolean; RFOpen output boolean; leftMotor input; rightMotor input; CLOSED input; CLOSING input; OPEN input; OPENING input; counter local uint8

== stateflow chart gate_V25_2016a/HardwareOutputWrapper/A_HardwareOutputWrapper_BT_KP_RF/MotorHandler/MotorsHandler ==
  state MonitorChange
  state UpdatePins
    (default) -> (junction 91) : /* updating motor Pins Switch case */
    (junction 91) -> (junction 92) [order 1] : [(leftMotor == OPENING) && ((rightMotor == CLOSED) || (rightMotor == OPEN))]
    (junction 92) -> (junction 100) : {LeftPin = true;...
        | ComPin = true;...
        | RightPin = false;}
    (junction 91) -> (junction 93) [order 2]
    (junction 93) -> (junction 94) [order 1] : [(leftMotor == CLOSING) && ((rightMotor == CLOSED) || (rightMotor == OPEN))]
    (junction 94) -> (junction 99) : {LeftPin = false;...
        | ComPin = false;...
        |  RightPin = true;}
    (junction 93) -> (junction 95) [order 2]
    (junction 95) -> (junction 96) [order 1] : [(rightMotor == CLOSING) && ((leftMotor == CLOSED) || (leftMotor == OPEN))]
    (junction 96) -> (junction 98) : {LeftPin = true;...
        | ComPin = false;...
        | RightPin = false;}
    (junction 95) -> (junction 102) [order 2]
    (junction 102) -> (junction 103) [order 1] : [(rightMotor == OPENING) && ((leftMotor == CLOSED) || (leftMotor == OPEN))]
    (junction 103) -> (junction 110) : {LeftPin = false;...
        | ComPin = true;...
        | RightPin = true;}
    (junction 102) -> (junction 104) [order 2]
    (junction 104) -> (junction 105) [order 1] : [(rightMotor == OPENING) && (leftMotor == OPENING)]
    (junction 105) -> (junction 111) : {LeftPin = true;...
        | ComPin = true;...
        | RightPin = true;}
    (junction 104) -> (junction 106) [order 2]
    (junction 106) -> (junction 107) [order 1] : [(rightMotor == CLOSING) && (leftMotor == CLOSING)]
    (junction 107) -> (junction 112) : {LeftPin = false;...
        | ComPin = false;...
        | RightPin = false;}
    (junction 106) -> (junction 123) [order 2]
    (junction 123) -> (junction 124) [order 1] : [((rightMotor == CLOSED) || (rightMotor == OPEN)) ...
        | && ((leftMotor == CLOSED) || (leftMotor == OPEN))]
    (junction 123) -> (junction 97) [order 2]
    (junction 124) -> (junction 125) : {LeftPin = false;...
        | ComPin = true;...
        | RightPin = false;}
    (junction 100) -> (junction 99)
    (junction 99) -> (junction 98)
    (junction 98) -> (junction 110)
    (junction 125) -> (junction 97)
    (junction 112) -> (junction 125)
    (junction 111) -> (junction 112)
    (junction 110) -> (junction 111)
    (junction 97) -> (junction 101)
  (default) -> MonitorChange
  UpdatePins -> MonitorChange
  MonitorChange -> UpdatePins : [(leftMotor != oldLeft) ...
      | || (rightMotor != oldRight)]
  data: LeftPin output =false; ComPin output =true; RightPin output =false; leftMotor input; oldLeft input; rightMotor input; oldRight input; CLOSED input; CLOSING input; OPEN input; OPENING input

== stateflow chart gate_V25_2016a/GateLogic/C_Variant_RF/GateLogicStatemachine ==
  state init
    entry:
    gotoReady = false;
    bulb = 0;
    leftMotor = CLOSED;
    rightMotor = CLOSED;
  state opening
    entry:
    bulb = true;
    state openLeftSide
      entry:
      leftMotor = OPENING;
      openSideDelay = 0;
      during:
      openSideDelay++;
    state openRightSide
      entry:
      rightMotor = OPENING;
    (default) -> openLeftSide
    openLeftSide -> openRightSide : [openSideDelay == OPEN_SIDE_VALUE]
  state ready
    entry:
    bulb = false;
    leftMotor = CLOSED;
    rightMotor = CLOSED;
    openingActive = 0;
    state openingGate
      entry:
      openingActive = OPENING_ACTIVE;
    state MonitorInput
    (default) -> MonitorInput
    MonitorInput -> openingGate [order 1] : [RfOpen]
    MonitorInput -> openingGate [order 2] : [passSwitch == true]
  state closing
    state closingRightSide
      entry:
      rightMotor = CLOSING;
      closeSideDelay = 0;
      during:
      closeSideDelay++;
    state closingLeftSide
      entry:
      leftMotor = CLOSING;
    (default) -> closingRightSide
    closingRightSide -> closingLeftSide : [closeSideDelay == CLOSE_SIDE_VALUE]
  state open
    state gateOpen
      entry:
      closing_active = false;
      leftMotor = OPEN;
      rightMotor = OPEN;
      openTimer = 0;
      du:
      openTimer++;
    state closing
      entry:
      closing_active = true;
    (default) -> gateOpen
    gateOpen -> open.closing [order 3] : [passSwitch == true]
    gateOpen -> open.closing [order 1] : [RfClose]
    gateOpen -> open.closing [order 2] : [openTimer == OPEN_TIMEOUT]
  (default) -> init
  ready -> opening : [openingActive == OPENING_ACTIVE]
  init -> ready
  closing -> ready : [(current_sensor == 0)...
      | &&(leftMotor == CLOSING)...
      | &&(rightMotor == CLOSING)]
  opening -> open : [(current_sensor == 0)...
      | && (leftMotor == OPENING)...
      | && (rightMotor == OPENING)]
  open -> closing : [closing_active == true]
  data: RfOpen input; openingActive local uint8; passSwitch input; password local uint8 size=6; trialPass local uint8 size=6; counter local uint8; closing_active local uint8; current_sensor input; initCounter local uint8; openSideDelay local uint16; leftMotor output uint8 =0; rightMotor output uint8 =0; bulb output boolean; RfClose input; closeSideDelay local uint16; OPENING_ACTIVE input =2; OPEN_SIDE_VALUE input =20; CLOSE_SIDE_VALUE input =20; OPEN_TIMEOUT input =999999; OPENING input =2; CLOSED input =1; CLOSING input =4; OPEN input =3; passAssigned output boolean; gotoReady local boolean; passSuccess output uint8 =0; passTimer local uint16; TIMEOUT input; openTimer local uint16

== stateflow chart gate_V25_2016a/EEPROM/EEPROM_Control ==
  state Idle
  state sendData
    entry:
    readReq = true;
  state Read
    entry:
    readReq = false;
  state write
    entry:
    writeReq = true;
  state clear
    entry:
    clearReq = true;
  Read -> sendData
  sendData -> Idle : [readComplete]/readReq = false;
  clear -> Idle [order 2] : [(hasChanged(passSw))...
      |  && (passSw == false)...
      | && (passAssigned == false)]
      | /clearReq = false;
  Idle -> clear : [(hasChanged(passSw))...
      |  && (passSw == true)]
  (default) -> Read
  write -> Read : [writeComplete]/writeReq = false;
  clear -> write [order 1] : [(hasChanged(passSw))...
      |  && (passSw == false)...
      | && (passAssigned == true)]
      | /clearReq = false;
  data: passSw input; passAssigned input; readComplete input; writeComplete input; clearReq output boolean =false; readReq output boolean =false; writeReq output boolean =false

== stateflow chart gate_V25_2016a/HardwareOutputWrapper/B_HardwareOutputWrapper_KP_RF/LedHandler/LedHandler ==
  state AssigningPass
    en:
    counter = 0;
    state Start
      en:
      yellowLedPin = true;
      greenLedPin = false;
      redLedPin = false;
    state correctPassAssigned
      du:
      counter++;
    state incorrectPassAssigned
      du:
      counter++;
    (default) -> AssigningPass.Start
    AssigningPass.Start -> correctPassAssigned [order 1] : [PassAssigned == true]/greenLedPin = true;
    AssigningPass.Start -> incorrectPassAssigned [order 2] : [(PassSw == false) && (PassAssigned == false)]
        | /redLedPin = true;...
        | yellowLedPin = false;
    correctPassAssigned -> correctPassAssigned : [(hasChanged(PassSw)) ...
        | && (PassSw == false)]
        | /yellowLedPin = false;
  state EnteringPass
    en:
    counter = 0;
    state correctPass
      en:
      yellowLedPin = false;
      greenLedPin = true;
      redLedPin = false;
      du:
      counter++;
    state Start
    state IncorrectPass
      en:
      yellowLedPin = false;
      greenLedPin = false;
      redLedPin = true;
      du:
      counter++;
    EnteringPass.Start -> correctPass [order 1] : [PassSuccess == PASSWORD_VERIFIED]
    (default) -> EnteringPass.Start
    EnteringPass.Start -> IncorrectPass [order 2] : [(PassSuccess == TIMEOUT)...
        |  || (PassSuccess == WRONG_PASSWORD)]
  state Idle
    en:
    yellowLedPin = false;
    greenLedPin = false;
    redLedPin = false;
  state GateOn
    en:
    yellowLedPin = false;
    greenLedPin = true;
    redLedPin = false;
  (default) -> Idle
  EnteringPass -> Idle [order 2] : [PassSuccess == NO_PASS_ASSIG]
  Idle -> AssigningPass [order 1] : [PassSw == true]
  correctPass -> Idle : [counter >= 4800]
  AssigningPass -> Idle [order 1] : [(counter >= 4900)]
  Idle -> EnteringPass [order 2] : [(hasChanged(KpCharPressed)) ...
      | && (KpCharPressed != 0)...
      | && (KpCharPressed != OPEN_CHAR)...
      | && (KpCharPressed != CLOSE_CHAR)...
      | && (PassAssigned == true)]
      | /yellowLedPin = true;
  IncorrectPass -> Idle : [counter >= 4800]
  Idle -> GateOn [order 3] : [(leftMotor == OPENING)...
      |  || (leftMotor == OPEN)...
      |  || (leftMotor == CLOSING)]
  GateOn -> Idle : [leftMotor == CLOSED]
  EnteringPass -> GateOn [order 1] : [(leftMotor == OPENING)...
      | || (leftMotor == OPEN)...
      | || (leftMotor == CLOSING)]
  AssigningPass -> GateOn [order 2] : [(leftMotor == OPENING)...
      |  || (leftMotor == OPEN)...
      |  || (leftMotor == CLOSING)]
  data: leftMotor input; rightMotor input; greenLedPin output boolean =false; redLedPin output boolean =false; yellowLedPin output boolean =false; PassSw input; counter local uint16; PassAssigned input; PassSuccess input; KpCharPressed input; CLOSED input; CLOSING input; OPEN input; OPENING input; OPENING_ACTIVE input; WRONG_PASSWORD input; PASSWORD_VERIFIED input; NO_PASS_ASSIG input; OPEN_CHAR input; CLOSE_CHAR input; TIMEOUT input

== stateflow chart gate_V25_2016a/HardwareOutputWrapper/B_HardwareOutputWrapper_KP_RF/MotorHandler/MotorsHandler ==
  state MonitorChange
  state UpdatePins
    (default) -> (junction 91) : /* updating motor Pins Switch case */
    (junction 91) -> (junction 92) [order 1] : [(leftMotor == OPENING) && ((rightMotor == CLOSED) || (rightMotor == OPEN))]
    (junction 92) -> (junction 100) : {LeftPin = true;...
        | ComPin = true;...
        | RightPin = false;}
    (junction 91) -> (junction 93) [order 2]
    (junction 93) -> (junction 94) [order 1] : [(leftMotor == CLOSING) && ((rightMotor == CLOSED) || (rightMotor == OPEN))]
    (junction 94) -> (junction 99) : {LeftPin = false;...
        | ComPin = false;...
        |  RightPin = true;}
    (junction 93) -> (junction 95) [order 2]
    (junction 95) -> (junction 96) [order 1] : [(rightMotor == CLOSING) && ((leftMotor == CLOSED) || (leftMotor == OPEN))]
    (junction 96) -> (junction 98) : {LeftPin = true;...
        | ComPin = false;...
        | RightPin = false;}
    (junction 95) -> (junction 102) [order 2]
    (junction 102) -> (junction 103) [order 1] : [(rightMotor == OPENING) && ((leftMotor == CLOSED) || (leftMotor == OPEN))]
    (junction 103) -> (junction 110) : {LeftPin = false;...
        | ComPin = true;...
        | RightPin = true;}
    (junction 102) -> (junction 104) [order 2]
    (junction 104) -> (junction 105) [order 1] : [(rightMotor == OPENING) && (leftMotor == OPENING)]
    (junction 105) -> (junction 111) : {LeftPin = true;...
        | ComPin = true;...
        | RightPin = true;}
    (junction 104) -> (junction 106) [order 2]
    (junction 106) -> (junction 107) [order 1] : [(rightMotor == CLOSING) && (leftMotor == CLOSING)]
    (junction 107) -> (junction 112) : {LeftPin = false;...
        | ComPin = false;...
        | RightPin = false;}
    (junction 106) -> (junction 123) [order 2]
    (junction 123) -> (junction 124) [order 1] : [((rightMotor == CLOSED) || (rightMotor == OPEN)) ...
        | && ((leftMotor == CLOSED) || (leftMotor == OPEN))]
    (junction 123) -> (junction 97) [order 2]
    (junction 124) -> (junction 125) : {LeftPin = false;...
        | ComPin = true;...
        | RightPin = false;}
    (junction 100) -> (junction 99)
    (junction 99) -> (junction 98)
    (junction 98) -> (junction 110)
    (junction 125) -> (junction 97)
    (junction 112) -> (junction 125)
    (junction 111) -> (junction 112)
    (junction 110) -> (junction 111)
    (junction 97) -> (junction 101)
  (default) -> MonitorChange
  UpdatePins -> MonitorChange
  MonitorChange -> UpdatePins : [(leftMotor != oldLeft) ...
      | || (rightMotor != oldRight)]
  data: LeftPin output =false; ComPin output =true; RightPin output =false; leftMotor input; oldLeft input; rightMotor input; oldRight input; CLOSED input; CLOSING input; OPEN input; OPENING input

== stateflow chart gate_V25_2016a/HardwareInputWrapper/HIL/currentSensorWrapperOld/SquareWaveDetector ==
  state Running
    entry:
    counterHigh = 0;
    counterLow= 0;
    currentValue = 1;
    state High
    state Low
    (default) -> High
    High -> High [order 2] : [CurrentAnalogIn > 1000]
        | /counterHigh++;
    High -> Low [order 1] : [CurrentAnalogIn < 1000]
    Low -> High [order 1] : [CurrentAnalogIn > 1000]
    Low -> Low [order 2] : [CurrentAnalogIn < 1000]
        | /counterLow++
  state Stop
    entry:
    currentValue = 0;
  (default) -> Stop
  Stop -> Running : [CurrentAnalogIn > 1000]
  Running -> Stop : [(counterHigh >= 200)...
      |  || (counterLow >= 200)]
  data: CurrentAnalogIn input; currentValue output uint8; counterHigh local uint16; counterLow local uint16
